simulink model "Q1"  (R2021b)
settings: Solver=VariableStepAuto  StartTime=0.0  StopTime=5  RelTol=1e-3
undefined symbols (not defined in the file or in its folder): H_x, H_y, Hds, Hfs, V_s
libraries: cstblocks x4, simulink x1
settings Model: Creator=user  LastModifiedBy=user

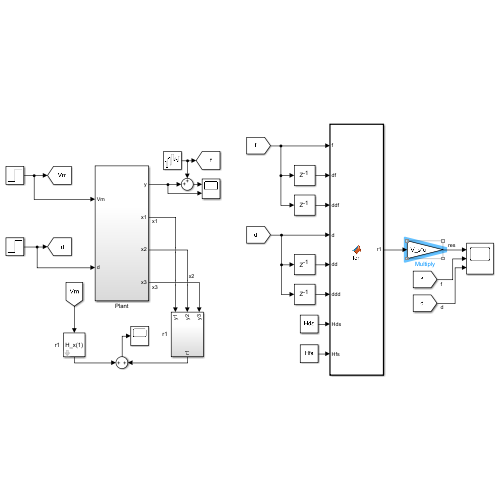
[thumbnail: Simulink's stored preview of the top-level diagram]
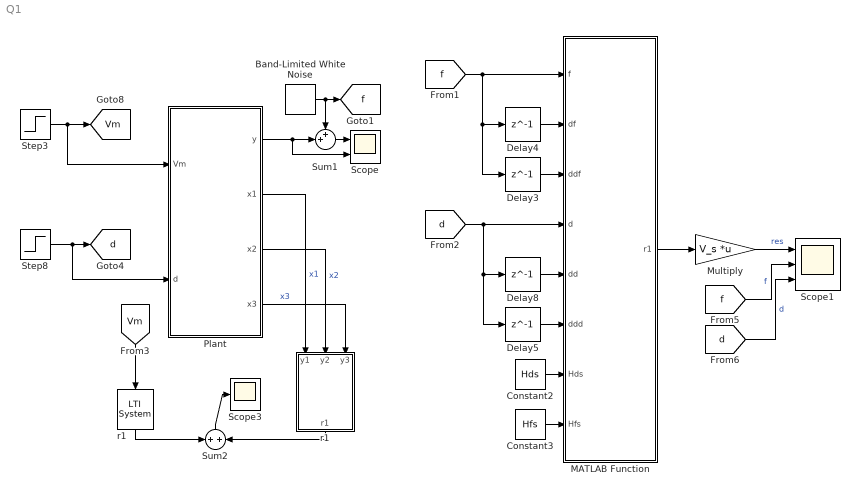
== system Q1 ==
  " r1" : Subsystem
  Band-Limited White Noise : simulink/Sources/Band-Limited White Noise  Cov=[2]  Ts=0.1  seed=[23341]
  Constant2 : Constant  Value=Hds
  Constant3 : Constant  Value=Hfs
  Delay{3..5,8} (4 alike) : Delay  DelayLength=1  InitialCondition=0
  MATLAB Function : MATLAB Function  TreatAsAtomicUnit=on
  Multiply : Gain  Gain=V_s  Multiplication=Matrix(K*u)
  Plant : Subsystem
  Scope : Scope  NumInputPorts=2
  Scope1 : Scope  NumInputPorts=3
  Scope3 : Scope
  Step3 : Step  Time=0  After=2  SampleTime=0
  Step8 : Step  After=0.1  SampleTime=0
  Sum1 : Sum  Inputs=++|
  Sum2 : Sum  Inputs=+|+
  r1 : cstblocks/LTI System  sys=H_x(1)  IC=[]
  tag scope: Vm=global, d=global, f=global
  wires:
  Step8/1 -> Plant/2(d), [d]
  Step3/1 -> Plant/1(Vm), [Vm]
  MATLAB Function/1(r1) -> Multiply/1
  [f] -> MATLAB Function/1(f), Delay3/1, Delay4/1
  Multiply/1 -> Scope1/1  "res"
  Delay4/1 -> MATLAB Function/2(df)
  Delay8/1 -> MATLAB Function/5(dd)
  Constant2/1 -> MATLAB Function/7(Hds)
  [f] -> Scope1/2  "f"
  Constant3/1 -> MATLAB Function/8(Hfs)
  Delay3/1 -> MATLAB Function/3(ddf)
  Delay5/1 -> MATLAB Function/6(ddd)
  [d] -> Scope1/3  "d"
  [d] -> Delay5/1, Delay8/1, MATLAB Function/4(d)
  Plant/1(y) -> Scope/2, Sum1/2
  Band-Limited White Noise/1 -> [f], Sum1/1
  Plant/3(x2) -> " r1"/2(y2)  "x2"
  Plant/4(x3) -> " r1"/3(y3)  "x3"
  Plant/2(x1) -> " r1"/1(y1)  "x1"
  Sum1/1 -> Scope/1
  [Vm] -> r1/1
  Sum2/1 -> Scope3/1
  r1/1 -> Sum2/1
  " r1"/1(r1) -> Sum2/2

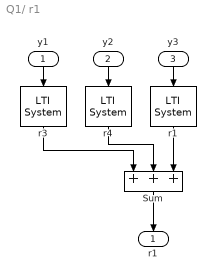
== system Q1/ r1 ==
  y1 : Inport
  y2 : Inport  Port=2
  y3 : Inport  Port=3
  " r1" : cstblocks/LTI System  sys=H_y(1,3)  IC=[]
  Sum : Sum  Inputs=+++
  r3 : cstblocks/LTI System  sys=H_y(1,1)  IC=[]
  r4 : cstblocks/LTI System  sys=H_y(1,2)  IC=[]
  r1 : Outport
  wires:
  y2/1 -> r4/1
  y1/1 -> r3/1
  y3/1 -> " r1"/1
  r3/1 -> Sum/1
  r4/1 -> Sum/2
  " r1"/1 -> Sum/3
  Sum/1 -> r1/1

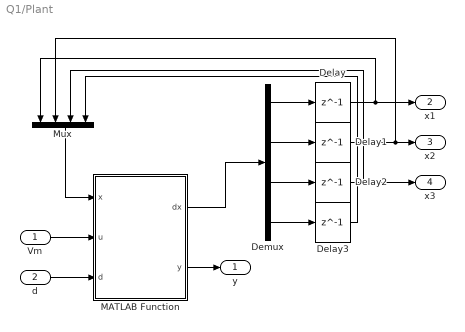
== system Q1/Plant ==
  Vm : Inport
  d : Inport  Port=2
  Delay{,1..3} (4 alike) : Delay  DelayLength=1  InputProcessing=Columns as channels (frame based)  SampleTime=0.1
  Demux : Demux
  MATLAB Function : MATLAB Function  TreatAsAtomicUnit=on
  Mux : Mux
  y : Outport
  x1 : Outport  Port=2
  x2 : Outport  Port=3
  x3 : Outport  Port=4
  wires:
  Vm/1 -> MATLAB Function/2(u)
  Mux/1 -> MATLAB Function/1(x)
  Demux/1 -> Delay/1
  Demux/2 -> Delay1/1
  Delay/1 -> Mux/1, x1/1
  Delay1/1 -> x2/1, Mux/2
  d/1 -> MATLAB Function/3(d)
  MATLAB Function/2(y) -> y/1
  MATLAB Function/1(dx) -> Demux/1
  Demux/4 -> Delay3/1
  Demux/3 -> Delay2/1
  Delay3/1 -> Mux/4
  Delay2/1 -> x3/1, Mux/3

== matlab function Q1/MATLAB Function ==
  data: f input; r1 output; df input; ddf input; d input; dd input; ddd input; Hds input; Hfs input
function r1 = fcn(f,df,ddf,d,dd,ddd,Hds,Hfs)
d=[ddd;dd;d];
f=[ddf;df;f];
r1 = (Hds*d + Hfs*f);

== matlab function Q1/Plant/MATLAB Function ==
  data: x input; u input; dx output; d input; y output
function [dx,y]  = plant(x,u,d)
% dx = zeros(2,1);
A=[1 0.0001125 -0.05685 8.174e-006;
    0 1.01 0.01162 0.03003;
    0 -0.00384 0.9441 -0.0002962;
    0 0.6434 0.768 1.005];
B=[0.005288 0.03723 -0.1792 2.461]';
Bd=B;
C=[eye(3) zeros(3,1)];
temp = A*x;
temp2 = B*u;
temp3 = Bd*d;
y=C*x;
dx = temp(:,1) + temp2(:,1) + temp3(:,1);
end
